simulink model "PulsoSqrtSumaR_6CV3"  (R2023a)
settings: Solver=VariableStepAuto  StartTime=0.0  StopTime=10  RelTol=1e-3
libraries: dspfdesign x1, dspxfrm3 x1
settings Model: Creator=bborj  LastModifiedBy=Jorge
settings SolverCC: AlgebraicLoopSolver=TrustRegion
settings DebuggingCC: UnconnectedInputMsg=warning  UnconnectedOutputMsg=warning  UnconnectedLineMsg=warning
settings ModelReferenceCC: EnableRefExpFcnMdlSchedulingChecks=on
settings RTWCC: DLArmComputeVersion=19.05

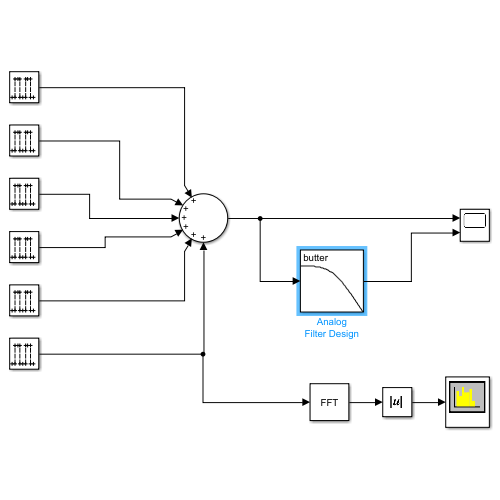
[thumbnail: Simulink's stored preview of the top-level diagram]
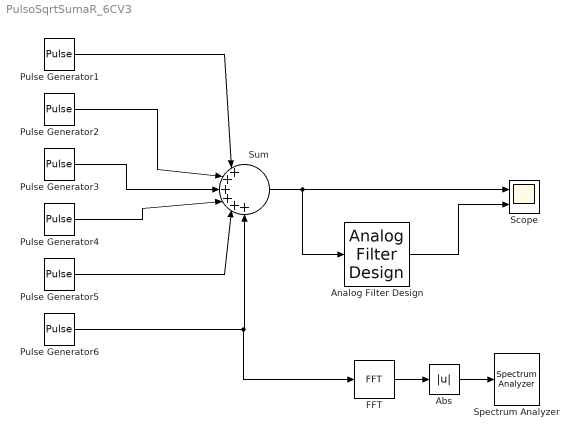
== system PulsoSqrtSumaR_6CV3 ==
  Abs : Abs  SaturateOnIntegerOverflow=off
  Analog Filter Design : dspfdesign/Analog Filter Design  method=Butterworth  filttype=Lowpass  N=1  Wlo=2*pi*1000  Whi=80  Rp=2  Rs=40
  FFT : dspxfrm3/FFT  FFTImplementation=Auto  CompMethod=Table lookup  TableOpt=NEW  TableOptActive=Speed  BitRevOrder=off  Normalize=off  InheritFFTLength=on  FFTLength=64  WrapInput=on  roundingMode=Floor  overflowMode=off  firstCoeffDataTypeStr=Inherit: Same word length as input  firstCoeffLastDataTypeStr=Inherit: Same word length as input  outputMin=[]  outputMax=[]
  Pulse Generator1 : DiscretePulseGenerator  Amplitude=4  Period=1024  PulseWidth=10  SampleTime=1/1000
  Pulse Generator2 : DiscretePulseGenerator  Amplitude=2  Period=1024  PulseWidth=10  PhaseDelay=10  SampleTime=1/1000
  Pulse Generator3 : DiscretePulseGenerator  Amplitude=-1  Period=1024  PulseWidth=10  PhaseDelay=20  SampleTime=1/1000
  Pulse Generator4 : DiscretePulseGenerator  Amplitude=-3  Period=1024  PulseWidth=10  PhaseDelay=30  SampleTime=1/1000
  Pulse Generator5 : DiscretePulseGenerator  Amplitude=2  Period=1024  PulseWidth=10  PhaseDelay=40  SampleTime=1/1000
  Pulse Generator6 : DiscretePulseGenerator  Amplitude=-4  Period=1024  PulseWidth=10  PhaseDelay=50  SampleTime=1/1000
  Scope : Scope  NumInputPorts=2
  Spectrum Analyzer : SpectrumAnalyzer  WindowPosition=[2882.000000,2.000000,958.000000,1048.000000,]  ScopeFrameLocation=window  SampleRate=1000  AxesScaling=Manual  Span=1000  StartFrequency=-500  StopFrequency=500  AveragingMethod=Exponential  YLimits=[-75.775909332143640995,14.302458552604326414]  DefaultConfigurationName=spbscopes.SpectrumAnalyzerBlockCfg  IsFrequencyInputMode=0  FrequencyVectorPort=0  FrequencyVectorFromPort=0  FrequencyInputRBWPort=0  FrequencyInputRBWFromPort=0
  Sum : Sum  Inputs=|++++++
  wires:
  Abs/1 -> Spectrum Analyzer/1
  FFT/1 -> Abs/1
  Pulse Generator6/1 -> FFT/1, Sum/6
  Pulse Generator1/1 -> Sum/1
  Pulse Generator2/1 -> Sum/2
  Pulse Generator5/1 -> Sum/5
  Pulse Generator3/1 -> Sum/3
  Pulse Generator4/1 -> Sum/4
  Sum/1 -> Analog Filter Design/1, Scope/1
  Analog Filter Design/1 -> Scope/2
